simulink model "TestingDynamics"  (R2019b)
settings: Solver=VariableStepAuto  StartTime=0.0  StopTime=10.0  RelTol=1e-3
values from neighbouring files (symbols this model uses):
  M_motor = [1, 1, 1, -1;             1, 1, -1, 1;             1, -1, -1, -1;             1, -1, 1, 1 ]    [HW7.m]
  tau2 = 0.015915    [HW7.m]
  V = 5    [HW7.m]
  V0 = 5    [HW7.m]
settings Model: Creator=cwhipp  LastModifiedBy=cwhipp

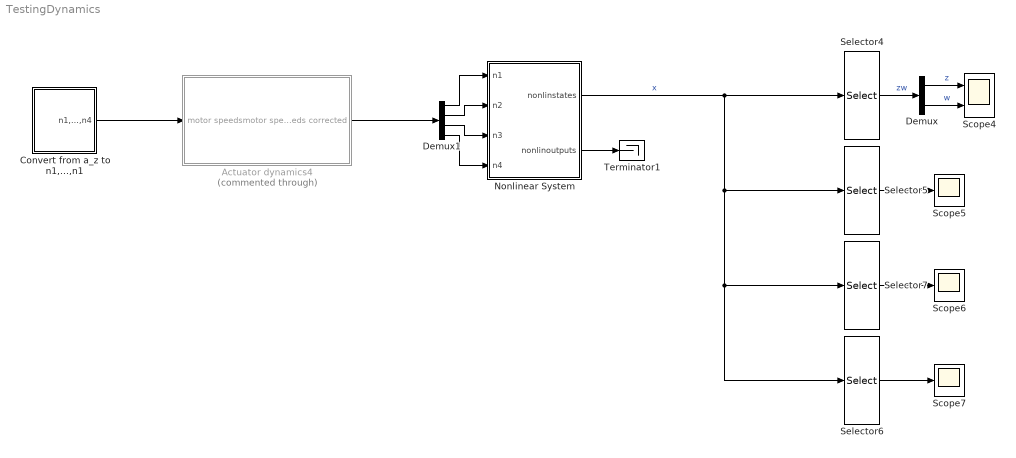
== system TestingDynamics ==
  Actuator dynamics4 : Subsystem  Commented=through
  Convert from a_z to n1,...,n1 : Subsystem
  Demux : Demux  Outputs=2
  Demux1 : Demux
  Nonlinear System : Subsystem
  Scope4 : Scope  NumInputPorts=2
  Scope5 : Scope
  Scope6 : Scope
  Scope7 : Scope
  Selector4 : Selector  InputPortWidth=12  IndexOptions=Index vector (dialog)  Indices=[1 2]  OutputSizes=1
  Selector5 : Selector  InputPortWidth=12  IndexOptions=Index vector (dialog)  Indices=[3 4 5 6]  OutputSizes=1
  Selector6 : Selector  InputPortWidth=12  IndexOptions=Index vector (dialog)  Indices=[11 12]  OutputSizes=1
  Selector7 : Selector  InputPortWidth=12  IndexOptions=Index vector (dialog)  Indices=[7 8 9 10]  OutputSizes=1
  Terminator1 : Terminator
  wires:
  Nonlinear System/1("nonlinstates ") -> Selector6/1, Selector7/1, Selector5/1, Selector4/1  "x"
  Selector5/1 -> Scope5/1
  Convert from a_z to n1,...,n1/1(n1,...,n4) -> Actuator dynamics4/1(motor speeds)
  Selector6/1 -> Scope7/1
  Selector7/1 -> Scope6/1
  Nonlinear System/2(nonlinoutputs) -> Terminator1/1
  Demux1/1 -> Nonlinear System/1("n1 ")
  Demux1/2 -> Nonlinear System/2(n2)
  Demux1/4 -> Nonlinear System/4(n4)
  Demux1/3 -> Nonlinear System/3(n3)
  Demux/2 -> Scope4/2  "w"
  Demux/1 -> Scope4/1  "z"
  Selector4/1 -> Demux/1  "zw"
  Actuator dynamics4/1(motor speeds corrected) -> Demux1/1

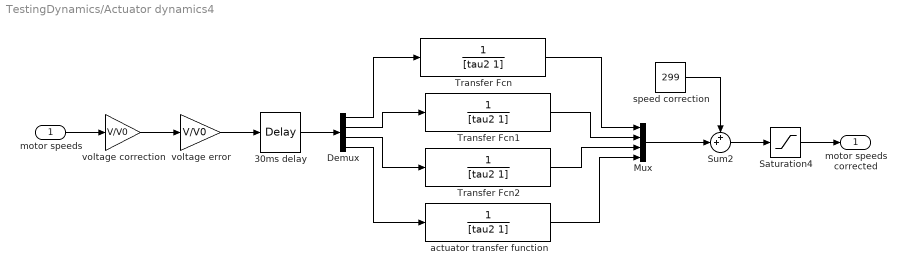
== system TestingDynamics/Actuator dynamics4 ==
  motor speeds : Inport
  30ms delay : TransportDelay  DelayTime=30e-3
  Demux : Demux
  Mux : Mux
  Saturation4 : Saturate  UpperLimit=500  LowerLimit=10
  Sum2 : Sum  Inputs=++|
  Transfer Fcn : TransferFcn  Denominator=[tau2 1]
  Transfer Fcn1 : TransferFcn  Denominator=[tau2 1]
  Transfer Fcn2 : TransferFcn  Denominator=[tau2 1]
  actuator transfer function : TransferFcn  Denominator=[tau2 1]
  speed correction : Constant  Value=299
  voltage correction : Gain  Gain=V/V0
  voltage error : Gain  Gain=V/V0
  motor speeds corrected : Outport
  wires:
  speed correction/1 -> Sum2/1
  voltage correction/1 -> voltage error/1
  Sum2/1 -> Saturation4/1
  Demux/2 -> Transfer Fcn1/1
  30ms delay/1 -> Demux/1
  Demux/4 -> actuator transfer function/1
  Demux/1 -> Transfer Fcn/1
  Demux/3 -> Transfer Fcn2/1
  voltage error/1 -> 30ms delay/1
  motor speeds/1 -> voltage correction/1
  Saturation4/1 -> motor speeds corrected/1
  Transfer Fcn/1 -> Mux/1
  Transfer Fcn1/1 -> Mux/2
  Transfer Fcn2/1 -> Mux/3
  actuator transfer function/1 -> Mux/4
  Mux/1 -> Sum2/2

== system TestingDynamics/Convert from a_z to n1,...,n1 ==
  Constant : Constant  Value=0
  Convert fom TEAR to n1,..,n4 : Gain  Gain=M_motor  Multiplication=Matrix(K*u)
  Mux : Mux
  Scope : Scope
  Step : Step  SampleTime=0
  n1,...,n4 : Outport
  wires:
  Convert fom TEAR to n1,..,n4/1 -> n1,...,n4/1
  Mux/1 -> Convert fom TEAR to n1,..,n4/1
  Step/1 -> Scope/1, Mux/1
  Constant/1 -> Mux/4, Mux/3, Mux/2

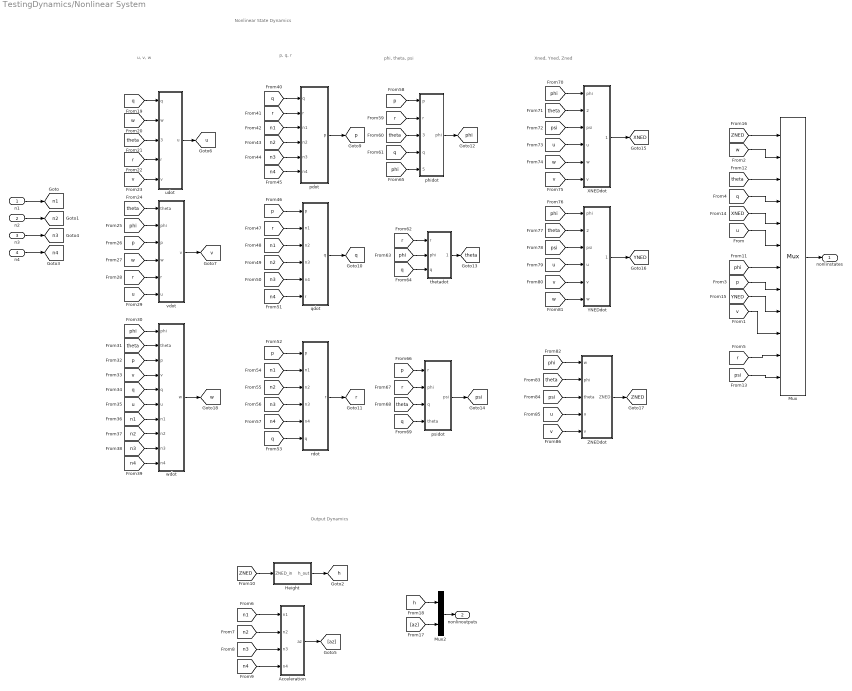
== system TestingDynamics/Nonlinear System ==
  note: Output Dynamics
  note: Nonlinear State Dynamics
  note: p, q, r
  note: u, v, w
  note: phi, theta, psi
  note: Xned, Yned, Zned
  "n1 " : Inport
  n2 : Inport  Port=2
  n3 : Inport  Port=3
  n4 : Inport  Port=4
  Acceleration : Subsystem
  Height : Subsystem
  Mux : Mux  Inputs=12
  Mux2 : Mux  Inputs=2
  "XNEDdot " : Subsystem
  "YNEDdot " : Subsystem
  ZNEDdot : Subsystem
  pdot : Subsystem
  phidot : Subsystem
  "psidot " : Subsystem
  qdot : Subsystem
  rdot : Subsystem
  "thetadot " : Subsystem
  udot : Subsystem
  vdot : Subsystem
  "wdot " : Subsystem
  "nonlinstates " : Outport
  nonlinoutputs : Outport  Port=2
  tag scope: XNED=global, YNED=global, ZNED=global, h=global, n1=global, n2=global, n3=global, n4=global, p=global, phi=global, psi=global, q=global, r=global, theta=global, u=global, v=global, w=global
  wires:
  [n2] -> Acceleration/2(n2)
  [n1] -> Acceleration/1(n1)
  [n3] -> Acceleration/3(n3)
  Acceleration/1(az) -> [az]
  [n4] -> Acceleration/4(n4)
  [ZNED] -> Height/1("ZNED_in ")
  Height/1("h_out ") -> [h]
  Mux/1 -> "nonlinstates "/1
  [h] -> Mux2/1
  [az] -> Mux2/2
  Mux2/1 -> nonlinoutputs/1
  udot/1("u ") -> [u]
  [q] -> udot/1("q ")
  [w] -> udot/2("w ")
  [theta] -> udot/3(theta)
  [r] -> udot/4("r ")
  [v] -> udot/5(v)
  "n1 "/1 -> [n1]
  n2/1 -> [n2]
  n3/1 -> [n3]
  n4/1 -> [n4]
  [theta] -> vdot/1(theta)
  [phi] -> vdot/2(phi)
  [p] -> vdot/3(p)
  [w] -> vdot/4(w)
  [r] -> vdot/5(r)
  [u] -> vdot/6(u)
  vdot/1(v) -> [v]
  [phi] -> "wdot "/1(phi)
  [theta] -> "wdot "/2(theta)
  [p] -> "wdot "/3(p)
  [v] -> "wdot "/4(v)
  [q] -> "wdot "/5(q)
  [u] -> "wdot "/6(u)
  [n1] -> "wdot "/7(n1)
  [n2] -> "wdot "/8(n2)
  [n3] -> "wdot "/9(n3)
  [n4] -> "wdot "/10(n4)
  "wdot "/1(w) -> [w]
  [n1] -> pdot/3(n1)
  [r] -> pdot/2(r)
  [n2] -> pdot/4(n2)
  [q] -> pdot/1(q)
  [n3] -> pdot/5(n3)
  [n4] -> pdot/6(n4)
  [p] -> qdot/1(p)
  [r] -> qdot/2(n1)
  [n1] -> qdot/3(n2)
  [n2] -> qdot/4(n3)
  [n3] -> qdot/5(n4)
  [n4] -> qdot/6(r)
  qdot/1(q) -> [q]
  [p] -> rdot/1(p)
  [n1] -> rdot/2(n1)
  [n2] -> rdot/3(n2)
  [n3] -> rdot/4(n3)
  [n4] -> rdot/5(n4)
  [q] -> rdot/6(q)
  rdot/1(r) -> [r]
  [p] -> phidot/1(p)
  [r] -> phidot/2(r)
  [theta] -> phidot/3(theta)
  [q] -> phidot/4(q)
  phidot/1(phi) -> [phi]
  [q] -> "thetadot "/3(q)
  [r] -> "thetadot "/1(r)
  [phi] -> "thetadot "/2(phi)
  "thetadot "/1(theta) -> [theta]
  pdot/1(p) -> [p]
  [phi] -> phidot/5(phi in)
  [r] -> "psidot "/2(phi)
  [p] -> "psidot "/1(r)
  [theta] -> "psidot "/3(q)
  [q] -> "psidot "/4(theta)
  "psidot "/1(psi) -> [psi]
  [phi] -> "XNEDdot "/1(phi)
  [u] -> "XNEDdot "/4(u)
  [w] -> "XNEDdot "/5(w)
  [v] -> "XNEDdot "/6(v)
  [theta] -> "XNEDdot "/2(theta)
  [psi] -> "XNEDdot "/3(psi)
  "XNEDdot "/1(XNED) -> [XNED]
  [w] -> "YNEDdot "/6(w)
  [v] -> "YNEDdot "/5(v)
  [u] -> "YNEDdot "/4(u)
  [psi] -> "YNEDdot "/3(psi)
  [theta] -> "YNEDdot "/2(theta)
  "YNEDdot "/1(YNED) -> [YNED]
  [phi] -> "YNEDdot "/1(phi)
  [phi] -> ZNEDdot/1(w)
  [theta] -> ZNEDdot/2(phi)
  [psi] -> ZNEDdot/3(theta)
  [u] -> ZNEDdot/4(u)
  [v] -> ZNEDdot/5(v)
  ZNEDdot/1(ZNED) -> [ZNED]
  [r] -> Mux/11
  [psi] -> Mux/12
  [phi] -> Mux/7
  [p] -> Mux/8
  [YNED] -> Mux/9
  [v] -> Mux/10
  [u] -> Mux/6
  [XNED] -> Mux/5
  [q] -> Mux/4
  [theta] -> Mux/3
  [w] -> Mux/2
  [ZNED] -> Mux/1

== system TestingDynamics/Nonlinear System/Acceleration ==
  n1 : Inport
  n2 : Inport  Port=2
  n3 : Inport  Port=3
  n4 : Inport  Port=4
  Gain : Gain  Gain=1.9060e-06
  Square{,1..3} (4 alike) : Math  Operator=square  SignedPower=off  SaturateOnIntegerOverflow=on
  Sum : Sum  Inputs=----
  az : Outport
  wires:
  n1/1 -> Square/1
  n2/1 -> Square1/1
  n3/1 -> Square2/1
  n4/1 -> Square3/1
  Square/1 -> Sum/1
  Square1/1 -> Sum/2
  Square2/1 -> Sum/3
  Square3/1 -> Sum/4
  Sum/1 -> Gain/1
  Gain/1 -> az/1

== system TestingDynamics/Nonlinear System/Height ==
  "ZNED_in " : Inport
  Gain : Gain  Gain=-1
  "h_out " : Outport
  wires:
  "ZNED_in "/1 -> Gain/1
  Gain/1 -> "h_out "/1

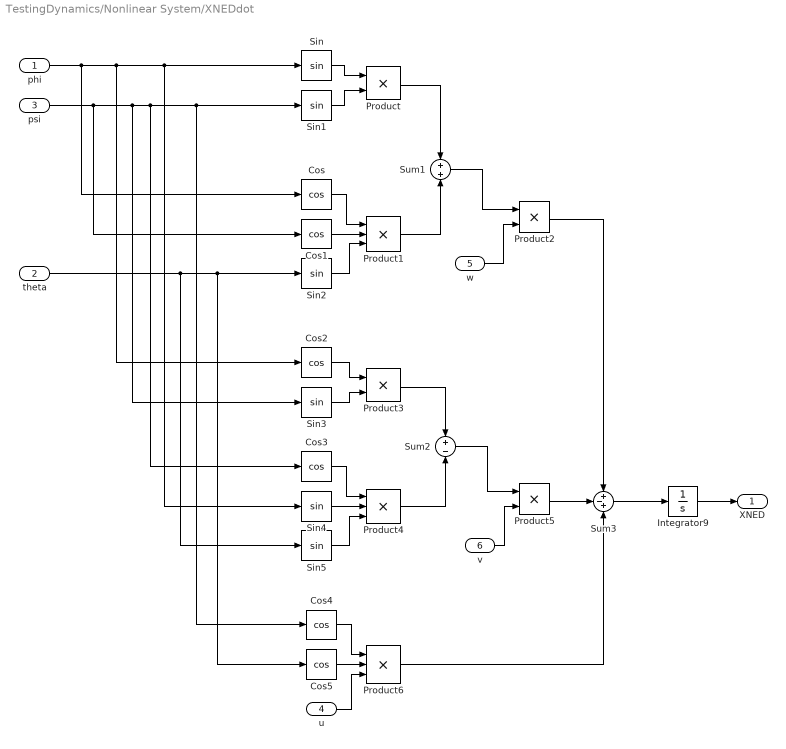
== system TestingDynamics/Nonlinear System/XNEDdot  ==
  phi : Inport
  theta : Inport  Port=2
  psi : Inport  Port=3
  u : Inport  Port=4
  w : Inport  Port=5
  v : Inport  Port=6
  Cos{,1..5} (6 alike) : Trigonometry  Operator=cos
  Integrator9 : Integrator
  Product{,2..3,5} (4 alike) : Product
  Product1 : Product  Inputs=3
  Product4 : Product  Inputs=3
  Product6 : Product  Inputs=3
  Sin{,1..5} (6 alike) : Trigonometry
  Sum1 : Sum
  Sum2 : Sum  Inputs=+-
  Sum3 : Sum  Inputs=+-+
  XNED : Outport
  wires:
  Cos1/1 -> Product1/2
  Sum1/1 -> Product2/1
  Product1/1 -> Sum1/2
  Product/1 -> Sum1/1
  Sin1/1 -> Product/2
  Sin/1 -> Product/1
  Cos/1 -> Product1/1
  Sin2/1 -> Product1/3
  w/1 -> Product2/2
  Product4/1 -> Sum2/2
  v/1 -> Product5/2
  Product3/1 -> Sum2/1
  Sum2/1 -> Product5/1
  Cos5/1 -> Product6/2
  u/1 -> Product6/3
  Product2/1 -> Sum3/1
  Product5/1 -> Sum3/2
  Product6/1 -> Sum3/3
  Sum3/1 -> Integrator9/1
  Integrator9/1 -> XNED/1
  Cos2/1 -> Product3/1
  Sin3/1 -> Product3/2
  Cos3/1 -> Product4/1
  phi/1 -> Cos2/1, Sin4/1, Sin/1, Cos/1
  Sin4/1 -> Product4/2
  Sin5/1 -> Product4/3
  psi/1 -> Cos1/1, Sin3/1, Cos3/1, Cos4/1, Sin1/1
  Cos4/1 -> Product6/1
  theta/1 -> Sin5/1, Cos5/1, Sin2/1

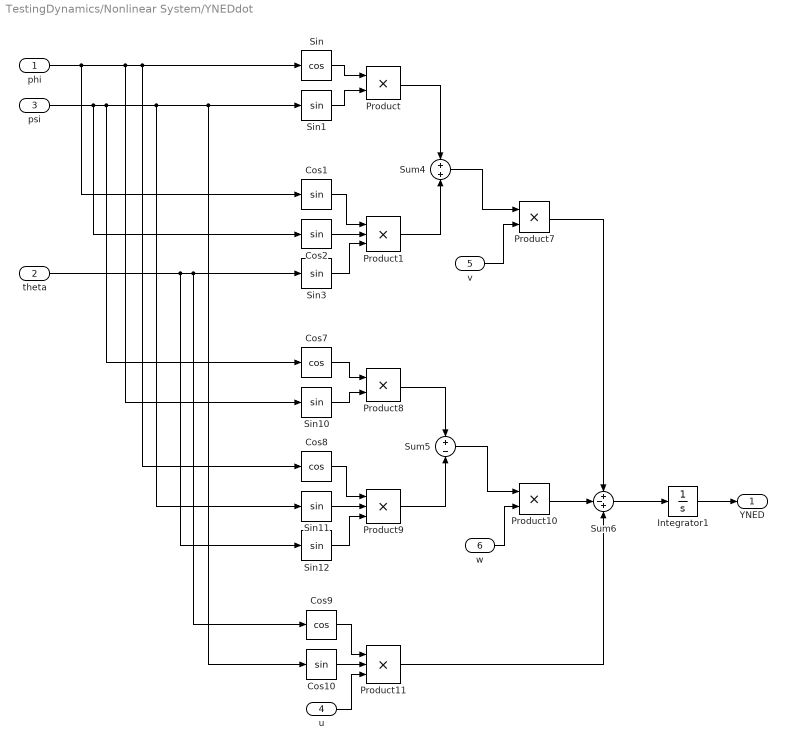
== system TestingDynamics/Nonlinear System/YNEDdot  ==
  phi : Inport
  theta : Inport  Port=2
  psi : Inport  Port=3
  u : Inport  Port=4
  v : Inport  Port=5
  w : Inport  Port=6
  Cos1 : Trigonometry
  Cos10 : Trigonometry
  Cos2 : Trigonometry
  Cos7 : Trigonometry  Operator=cos
  Cos8 : Trigonometry  Operator=cos
  Cos9 : Trigonometry  Operator=cos
  Integrator1 : Integrator
  Product{,7..8,10} (4 alike) : Product
  Product1 : Product  Inputs=3
  Product11 : Product  Inputs=3
  Product9 : Product  Inputs=3
  Sin : Trigonometry  Operator=cos
  Sin{1,3,10..12} (5 alike) : Trigonometry
  Sum4 : Sum
  Sum5 : Sum  Inputs=+-
  Sum6 : Sum  Inputs=+-+
  YNED : Outport
  wires:
  Sin/1 -> Product/1
  Cos7/1 -> Product8/1
  Sin11/1 -> Product9/2
  Sin12/1 -> Product9/3
  Product9/1 -> Sum5/2
  Sin10/1 -> Product8/2
  Sum5/1 -> Product10/1
  Product11/1 -> Sum6/3
  Sum6/1 -> Integrator1/1
  Product8/1 -> Sum5/1
  Product10/1 -> Sum6/2
  Product7/1 -> Sum6/1
  Sin3/1 -> Product1/3
  Cos1/1 -> Product1/1
  Product/1 -> Sum4/1
  Product1/1 -> Sum4/2
  Cos2/1 -> Product1/2
  v/1 -> Product7/2
  Cos9/1 -> Product11/1
  theta/1 -> Sin12/1, Cos9/1, Sin3/1
  Sin1/1 -> Product/2
  Sum4/1 -> Product7/1
  u/1 -> Product11/3
  w/1 -> Product10/2
  phi/1 -> Sin10/1, Cos8/1, Sin/1, Cos1/1
  psi/1 -> Cos2/1, Cos7/1, Sin11/1, Cos10/1, Sin1/1
  Cos8/1 -> Product9/1
  Integrator1/1 -> YNED/1
  Cos10/1 -> Product11/2

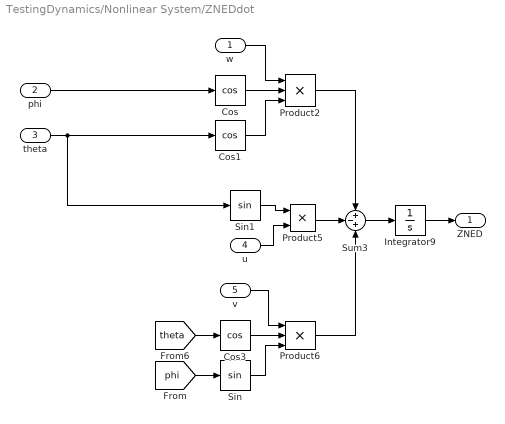
== system TestingDynamics/Nonlinear System/ZNEDdot ==
  w : Inport
  phi : Inport  Port=2
  theta : Inport  Port=3
  u : Inport  Port=4
  v : Inport  Port=5
  Cos : Trigonometry  Operator=cos
  Cos1 : Trigonometry  Operator=cos
  Cos3 : Trigonometry  Operator=cos
  Integrator9 : Integrator
  Product2 : Product  Inputs=3
  Product5 : Product
  Product6 : Product  Inputs=3
  Sin : Trigonometry
  Sin1 : Trigonometry
  Sum3 : Sum  Inputs=+-+
  ZNED : Outport
  wires:
  Product6/1 -> Sum3/3
  [phi] -> Sin/1
  Sum3/1 -> Integrator9/1
  Product2/1 -> Sum3/1
  Product5/1 -> Sum3/2
  u/1 -> Product5/2
  Integrator9/1 -> ZNED/1
  theta/1 -> Cos1/1, Sin1/1
  Cos/1 -> Product2/2
  Cos1/1 -> Product2/3
  Sin1/1 -> Product5/1
  phi/1 -> Cos/1
  [theta] -> Cos3/1
  w/1 -> Product2/1
  Cos3/1 -> Product6/2
  Sin/1 -> Product6/3
  v/1 -> Product6/1

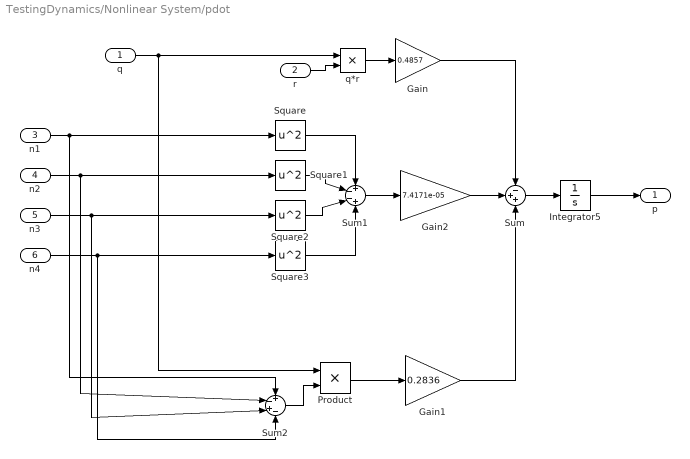
== system TestingDynamics/Nonlinear System/pdot ==
  q : Inport
  r : Inport  Port=2
  n1 : Inport  Port=3
  n2 : Inport  Port=4
  n3 : Inport  Port=5
  n4 : Inport  Port=6
  Gain : Gain  Gain=0.4857
  Gain1 : Gain  Gain=0.2836
  Gain2 : Gain  Gain=7.4171e-05
  Integrator5 : Integrator
  Product : Product
  Square{,1..3} (4 alike) : Math  Operator=square  SignedPower=off  SaturateOnIntegerOverflow=on
  Sum : Sum  Inputs=-++
  Sum1 : Sum  Inputs=+--+
  Sum2 : Sum  Inputs=+-+-
  q*r : Product
  p : Outport
  wires:
  Square1/1 -> Sum1/2
  Sum/1 -> Integrator5/1
  Square2/1 -> Sum1/3
  Square/1 -> Sum1/1
  Integrator5/1 -> p/1
  Square3/1 -> Sum1/4
  r/1 -> q*r/2
  q*r/1 -> Gain/1
  Sum1/1 -> Gain2/1
  Sum2/1 -> Product/2
  Product/1 -> Gain1/1
  Gain1/1 -> Sum/3
  n1/1 -> Sum2/1, Square/1
  n4/1 -> Square3/1, Sum2/4
  n3/1 -> Square2/1, Sum2/3
  n2/1 -> Sum2/2, Square1/1
  q/1 -> Product/1, q*r/1
  Gain/1 -> Sum/1
  Gain2/1 -> Sum/2

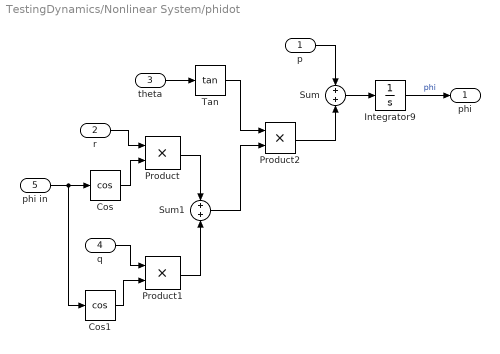
== system TestingDynamics/Nonlinear System/phidot ==
  p : Inport
  r : Inport  Port=2
  theta : Inport  Port=3
  q : Inport  Port=4
  phi in : Inport  Port=5
  Cos : Trigonometry  Operator=cos
  Cos1 : Trigonometry  Operator=cos
  Integrator9 : Integrator
  Product : Product
  Product1 : Product
  Product2 : Product
  Sum : Sum
  Sum1 : Sum
  Tan : Trigonometry  Operator=tan
  phi : Outport
  wires:
  Integrator9/1 -> phi/1  "phi"
  theta/1 -> Tan/1
  p/1 -> Sum/1
  q/1 -> Product1/1
  r/1 -> Product/1
  Cos/1 -> Product/2
  Product/1 -> Sum1/1
  Product1/1 -> Sum1/2
  Tan/1 -> Product2/1
  Sum1/1 -> Product2/2
  Product2/1 -> Sum/2
  Sum/1 -> Integrator9/1
  Cos1/1 -> Product1/2
  phi in/1 -> Cos1/1, Cos/1

== system TestingDynamics/Nonlinear System/psidot  ==
  r : Inport
  phi : Inport  Port=2
  q : Inport  Port=3
  theta : Inport  Port=4
  1/cos(theta) : Fcn  Expr=1/cos(u)
  Cos : Trigonometry  Operator=cos
  Integrator9 : Integrator
  Product : Product
  Product1 : Product
  Product2 : Product
  Sin : Trigonometry
  Sum1 : Sum
  psi : Outport
  wires:
  q/1 -> Product1/1
  Cos/1 -> Product/2
  Product1/1 -> Sum1/2
  Integrator9/1 -> psi/1
  Sin/1 -> Product1/2
  Product/1 -> Sum1/1
  r/1 -> Product/1
  Sum1/1 -> Product2/1
  theta/1 -> 1/cos(theta)/1
  1/cos(theta)/1 -> Product2/2
  Product2/1 -> Integrator9/1
  phi/1 -> Sin/1, Cos/1

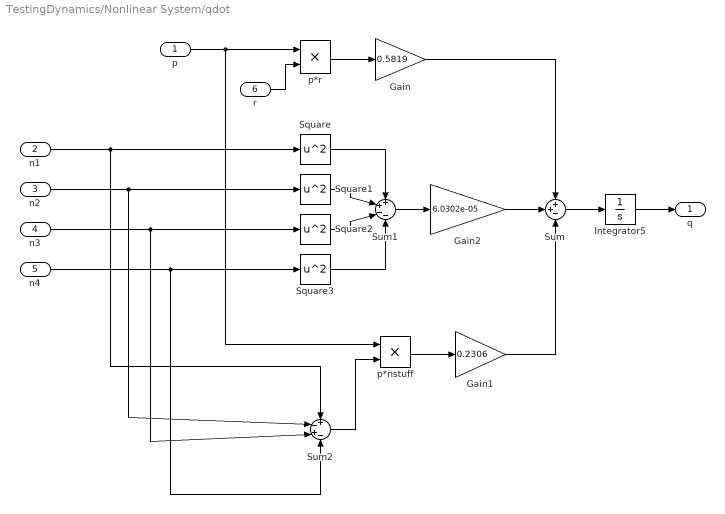
== system TestingDynamics/Nonlinear System/qdot ==
  p : Inport
  n1 : Inport  Port=2
  n2 : Inport  Port=3
  n3 : Inport  Port=4
  n4 : Inport  Port=5
  r : Inport  Port=6
  Gain : Gain  Gain=0.5819
  Gain1 : Gain  Gain=0.2306
  Gain2 : Gain  Gain=6.0302e-05
  Integrator5 : Integrator
  Square{,1..3} (4 alike) : Math  Operator=square  SignedPower=off  SaturateOnIntegerOverflow=on
  Sum : Sum  Inputs=++-
  Sum1 : Sum  Inputs=++--
  Sum2 : Sum  Inputs=+-+-
  p*nstuff : Product
  p*r : Product
  q : Outport
  wires:
  Sum/1 -> Integrator5/1
  Gain1/1 -> Sum/3
  n2/1 -> Sum2/2, Square1/1
  r/1 -> p*r/2
  Square3/1 -> Sum1/4
  Square1/1 -> Sum1/2
  p*nstuff/1 -> Gain1/1
  Integrator5/1 -> q/1
  p*r/1 -> Gain/1
  Square/1 -> Sum1/1
  Sum1/1 -> Gain2/1
  Square2/1 -> Sum1/3
  Sum2/1 -> p*nstuff/2
  Gain2/1 -> Sum/2
  Gain/1 -> Sum/1
  n4/1 -> Square3/1, Sum2/4
  n1/1 -> Sum2/1, Square/1
  n3/1 -> Square2/1, Sum2/3
  p/1 -> p*nstuff/1, p*r/1

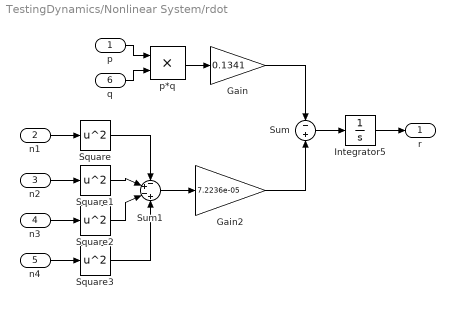
== system TestingDynamics/Nonlinear System/rdot ==
  p : Inport
  n1 : Inport  Port=2
  n2 : Inport  Port=3
  n3 : Inport  Port=4
  n4 : Inport  Port=5
  q : Inport  Port=6
  Gain : Gain  Gain=0.1341
  Gain2 : Gain  Gain=7.2236e-05
  Integrator5 : Integrator
  Square{,1..3} (4 alike) : Math  Operator=square  SignedPower=off  SaturateOnIntegerOverflow=on
  Sum : Sum  Inputs=-+
  Sum1 : Sum  Inputs=-+-+
  p*q : Product
  r : Outport
  wires:
  n3/1 -> Square2/1
  Gain/1 -> Sum/1
  n4/1 -> Square3/1
  q/1 -> p*q/2
  Square/1 -> Sum1/1
  p*q/1 -> Gain/1
  Square1/1 -> Sum1/2
  Sum/1 -> Integrator5/1
  p/1 -> p*q/1
  n2/1 -> Square1/1
  n1/1 -> Square/1
  Sum1/1 -> Gain2/1
  Square2/1 -> Sum1/3
  Square3/1 -> Sum1/4
  Gain2/1 -> Sum/2
  Integrator5/1 -> r/1

== system TestingDynamics/Nonlinear System/thetadot  ==
  r : Inport
  phi : Inport  Port=2
  q : Inport  Port=3
  Cos : Trigonometry  Operator=cos
  Integrator9 : Integrator
  Product : Product
  Product1 : Product
  Sin : Trigonometry
  Sum1 : Sum  Inputs=+-
  theta : Outport
  wires:
  Cos/1 -> Product/2
  r/1 -> Product1/1
  Product1/1 -> Sum1/2
  Integrator9/1 -> theta/1  "theta"
  Sin/1 -> Product1/2
  Product/1 -> Sum1/1
  q/1 -> Product/1
  Sum1/1 -> Integrator9/1
  phi/1 -> Sin/1, Cos/1

== system TestingDynamics/Nonlinear System/udot ==
  "q " : Inport
  "w " : Inport  Port=2
  theta : Inport  Port=3
  "r " : Inport  Port=4
  v : Inport  Port=5
  Gain : Gain  Gain=9.81
  Integrator5 : Integrator
  Sin : Trigonometry
  Sum : Sum  Inputs=+--
  q*w : Product
  r*v : Product
  "u " : Outport
  wires:
  Integrator5/1 -> "u "/1  "u"
  "q "/1 -> q*w/1
  "w "/1 -> q*w/2
  q*w/1 -> Sum/1
  theta/1 -> Sin/1
  Sin/1 -> Gain/1
  Gain/1 -> Sum/2
  "r "/1 -> r*v/1
  v/1 -> r*v/2
  r*v/1 -> Sum/3
  Sum/1 -> Integrator5/1

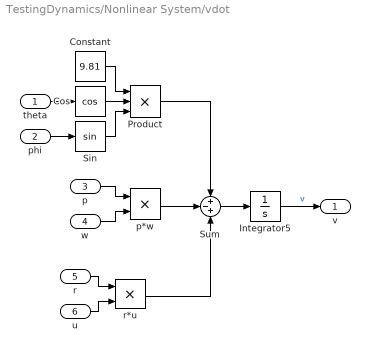
== system TestingDynamics/Nonlinear System/vdot ==
  theta : Inport
  phi : Inport  Port=2
  p : Inport  Port=3
  w : Inport  Port=4
  r : Inport  Port=5
  u : Inport  Port=6
  Constant : Constant  Value=9.81  SampleTime=0.05
  Cos : Trigonometry  Operator=cos
  Integrator5 : Integrator
  Product : Product  Inputs=3
  Sin : Trigonometry
  Sum : Sum  Inputs=+-+
  p*w : Product
  r*u : Product
  v : Outport
  wires:
  r/1 -> r*u/1
  p/1 -> p*w/1
  Sum/1 -> Integrator5/1
  Integrator5/1 -> v/1  "v"
  w/1 -> p*w/2
  u/1 -> r*u/2
  r*u/1 -> Sum/3
  theta/1 -> Cos/1
  Cos/1 -> Product/2
  Sin/1 -> Product/3
  phi/1 -> Sin/1
  Product/1 -> Sum/1
  p*w/1 -> Sum/2
  Constant/1 -> Product/1

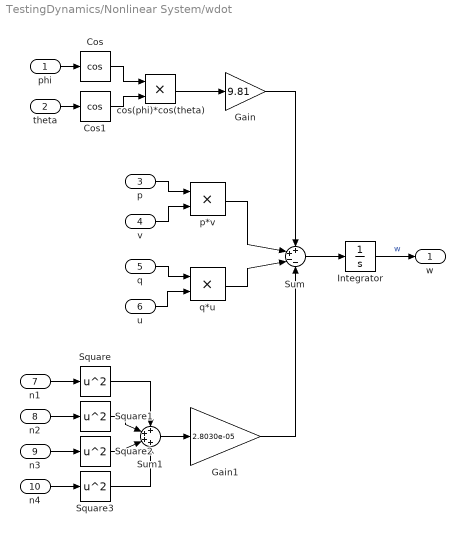
== system TestingDynamics/Nonlinear System/wdot  ==
  phi : Inport
  theta : Inport  Port=2
  p : Inport  Port=3
  v : Inport  Port=4
  q : Inport  Port=5
  u : Inport  Port=6
  n1 : Inport  Port=7
  n2 : Inport  Port=8
  n3 : Inport  Port=9
  n4 : Inport  Port=10
  Cos : Trigonometry  Operator=cos
  Cos1 : Trigonometry  Operator=cos
  Gain : Gain  Gain=9.81
  Gain1 : Gain  Gain=2.8030e-05
  Integrator : Integrator
  Square{,1..3} (4 alike) : Math  Operator=square  SignedPower=off  SaturateOnIntegerOverflow=on
  Sum : Sum  Inputs=++--
  Sum1 : Sum  Inputs=++++
  cos(phi)*cos(theta) : Product
  p*v : Product
  q*u : Product
  w : Outport
  wires:
  q*u/1 -> Sum/3
  u/1 -> q*u/2
  Integrator/1 -> w/1  "w"
  Gain/1 -> Sum/1
  q/1 -> q*u/1
  Sum/1 -> Integrator/1
  v/1 -> p*v/2
  p/1 -> p*v/1
  p*v/1 -> Sum/2
  theta/1 -> Cos1/1
  Cos1/1 -> cos(phi)*cos(theta)/2
  Cos/1 -> cos(phi)*cos(theta)/1
  cos(phi)*cos(theta)/1 -> Gain/1
  phi/1 -> Cos/1
  n1/1 -> Square/1
  Gain1/1 -> Sum/4
  Square/1 -> Sum1/1
  n2/1 -> Square1/1
  n3/1 -> Square2/1
  n4/1 -> Square3/1
  Square1/1 -> Sum1/2
  Square2/1 -> Sum1/3
  Square3/1 -> Sum1/4
  Sum1/1 -> Gain1/1
